simulink model "hireAdnFireV3"  (R2016b)
settings: Solver=ode4  StartTime=0.0  StopTime=1000.0  FixedStep=0.01  RelTol=1e-3
settings Model: Creator=Thomas  LastModifiedBy=Thomas

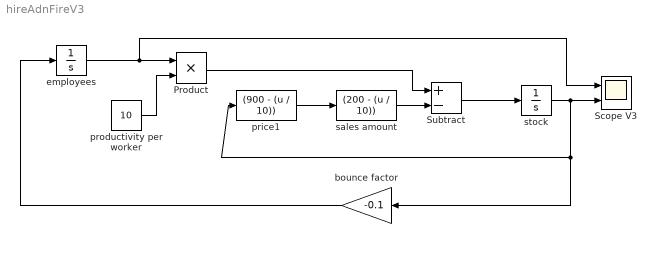
== system hireAdnFireV3 ==
  Product : Product
  Scope V3 : Scope  NumInputPorts=2
  Subtract : Sum  Inputs=+-
  bounce factor : Gain  Gain=-0.1
  employees : Integrator  InitialCondition=50
  price1 : Fcn  Expr=(900 - (u / 10))
  productivity per worker : Constant  Value=10
  sales amount : Fcn  Expr=(200 - (u / 10))
  stock : Integrator
  wires:
  productivity per worker/1 -> Product/2
  employees/1 -> Scope V3/1, Product/1
  stock/1 -> bounce factor/1, price1/1, Scope V3/2
  bounce factor/1 -> employees/1
  price1/1 -> sales amount/1
  Subtract/1 -> stock/1
  sales amount/1 -> Subtract/2
  Product/1 -> Subtract/1
